simulink model "case5"  (R2024b)
settings: Solver=FixedStepAuto  StartTime=0  StopTime=1  FixedStep=1e-7  RelTol=1e-3
values from neighbouring files (symbols this model uses):
  SG_D_1_D = 0.01056    [IEEE9_case_parameters.m]    (also in case1_parameters.m; case2_parameters.m; case3_parameters.m; case4_parameters.m)
  SG_D_1_EnableSaturation = 0    [IEEE9_case_parameters.m]    (also in case1_parameters.m; case2_parameters.m; case3_parameters.m; case4_parameters.m)
  SG_D_1_f0 = 60    [IEEE9_case_parameters.m]    (also in case1_parameters.m; case2_parameters.m; case3_parameters.m; case4_parameters.m)
  SG_D_1_H = 7.5    [IEEE9_case_parameters.m]    (also in case1_parameters.m; case2_parameters.m; case3_parameters.m; case4_parameters.m)
  SG_D_1_K_A = 20    [IEEE9_case_parameters.m]    (also in case1_parameters.m; case2_parameters.m; case3_parameters.m; case4_parameters.m)
  SG_D_1_K_E = 1.000000e+1    (= 10)    [IEEE9_case_parameters.m]    (also in case1_parameters.m; case2_parameters.m; case3_parameters.m; case4_parameters.m)
  SG_D_1_K_F = 2.363    [IEEE9_case_parameters.m]    (also in case1_parameters.m; case2_parameters.m; case3_parameters.m; case4_parameters.m)
  SG_D_1_K_s = 0.5    [IEEE9_case_parameters.m]    (also in case1_parameters.m = 5; case2_parameters.m = 5; case3_parameters.m = 5; case4_parameters.m = 5)
  SG_D_1_R_a = 0.001088    [IEEE9_case_parameters.m]    (also in case1_parameters.m; case2_parameters.m; case3_parameters.m; case4_parameters.m)
  SG_D_1_S_A = 1    [IEEE9_case_parameters.m]    (also in case1_parameters.m; case2_parameters.m; case3_parameters.m; case4_parameters.m)
  SG_D_1_S_B = 0.103    [IEEE9_case_parameters.m]    (also in case1_parameters.m; case2_parameters.m; case3_parameters.m; case4_parameters.m)
  SG_D_1_S_N = 10.659857    [IEEE9_case_parameters.m]    (also in case1_parameters.m; case2_parameters.m; case3_parameters.m; case4_parameters.m)
  SG_D_1_SpeedPara = 200    [IEEE9_case_parameters.m]    (also in case1_parameters.m; case2_parameters.m; case3_parameters.m; case4_parameters.m)
  SG_D_1_T_0 = 0.720173    [IEEE9_case_parameters.m]    (also in case1_parameters.m = 0.755522; case2_parameters.m = 0.808931; case3_parameters.m = 0.869402; case4_parameters.m = 0.729316)
  SG_D_1_T_1 = 0.3    [IEEE9_case_parameters.m]    (also in case1_parameters.m; case2_parameters.m; case3_parameters.m; case4_parameters.m)
  SG_D_1_T_2 = 0.05    [IEEE9_case_parameters.m]    (also in case1_parameters.m; case2_parameters.m; case3_parameters.m; case4_parameters.m)
  SG_D_1_T_3 = 0.02    [IEEE9_case_parameters.m]    (also in case1_parameters.m; case2_parameters.m; case3_parameters.m; case4_parameters.m)
  SG_D_1_T_4 = 0.005    [IEEE9_case_parameters.m]    (also in case1_parameters.m; case2_parameters.m; case3_parameters.m; case4_parameters.m)
  SG_D_1_T_A = 0.02    [IEEE9_case_parameters.m]    (also in case1_parameters.m; case2_parameters.m; case3_parameters.m; case4_parameters.m)
  SG_D_1_T_dd = 8.000000e+0    (= 8)    [IEEE9_case_parameters.m]    (also in case1_parameters.m; case2_parameters.m; case3_parameters.m; case4_parameters.m)
  SG_D_1_T_ddd = 0.04    [IEEE9_case_parameters.m]    (also in case1_parameters.m; case2_parameters.m; case3_parameters.m; case4_parameters.m)
  SG_D_1_T_E = 0.314    [IEEE9_case_parameters.m]    (also in case1_parameters.m; case2_parameters.m; case3_parameters.m; case4_parameters.m)
  SG_D_1_T_F = 0.35    [IEEE9_case_parameters.m]    (also in case1_parameters.m; case2_parameters.m; case3_parameters.m; case4_parameters.m)
  SG_D_1_T_qd = 0.8    [IEEE9_case_parameters.m]    (also in case1_parameters.m; case2_parameters.m; case3_parameters.m; case4_parameters.m)
  SG_D_1_T_qdd = 0.02    [IEEE9_case_parameters.m]    (also in case1_parameters.m; case2_parameters.m; case3_parameters.m; case4_parameters.m)
  SG_D_1_T_speed = 0.1    [IEEE9_case_parameters.m]    (also in case1_parameters.m = 200; case2_parameters.m = 200; case3_parameters.m = 200; case4_parameters.m = 200)
  SG_D_1_T_w = 0.5    [IEEE9_case_parameters.m]    (also in case1_parameters.m; case2_parameters.m; case3_parameters.m; case4_parameters.m)
  SG_D_1_V_ref = 1.990276    [IEEE9_case_parameters.m]    (also in case1_parameters.m = 2.042296; case2_parameters.m = 2.051388; case3_parameters.m = 2.089584; case4_parameters.m = 2.01845)
  SG_D_1_w_ref = 376.991118    [IEEE9_case_parameters.m]    (also in case1_parameters.m; case2_parameters.m; case3_parameters.m; case4_parameters.m)
  SG_D_1_wb = 6.000000e+1    (= 60)    [IEEE9_case_parameters.m]    (also in case1_parameters.m; case2_parameters.m; case3_parameters.m; case4_parameters.m)
  SG_D_1_x_d = 1.9    [IEEE9_case_parameters.m]    (also in case1_parameters.m; case2_parameters.m; case3_parameters.m; case4_parameters.m)
  SG_D_1_x_dd = 0.302    [IEEE9_case_parameters.m]    (also in case1_parameters.m; case2_parameters.m; case3_parameters.m; case4_parameters.m)
  SG_D_1_x_ddd = 0.204    [IEEE9_case_parameters.m]    (also in case1_parameters.m; case2_parameters.m; case3_parameters.m; case4_parameters.m)
  SG_D_1_x_l = 0.05    [IEEE9_case_parameters.m]    (also in case1_parameters.m; case2_parameters.m; case3_parameters.m; case4_parameters.m)
  SG_D_1_x_q = 1.3    [IEEE9_case_parameters.m]    (also in case1_parameters.m; case2_parameters.m; case3_parameters.m; case4_parameters.m)
  SG_D_1_x_qd = 0.5    [IEEE9_case_parameters.m]    (also in case1_parameters.m; case2_parameters.m; case3_parameters.m; case4_parameters.m)
  SG_D_1_x_qdd = 0.3    [IEEE9_case_parameters.m]    (also in case1_parameters.m; case2_parameters.m; case3_parameters.m; case4_parameters.m)
  SG_D_2_D = 0.02    [IEEE9_case_parameters.m]    (also in case1_parameters.m; case2_parameters.m; case3_parameters.m; case4_parameters.m)
  SG_D_2_EnableSaturation = 0    [IEEE9_case_parameters.m]    (also in case1_parameters.m; case2_parameters.m; case3_parameters.m; case4_parameters.m)
  SG_D_2_f0 = 60    [IEEE9_case_parameters.m]    (also in case1_parameters.m; case2_parameters.m; case3_parameters.m; case4_parameters.m)
  SG_D_2_H = 8.000000e+0    (= 8)    [IEEE9_case_parameters.m]    (also in case1_parameters.m; case2_parameters.m; case3_parameters.m; case4_parameters.m)
  SG_D_2_K_A = 20    [IEEE9_case_parameters.m]    (also in case1_parameters.m; case2_parameters.m; case3_parameters.m; case4_parameters.m)
  SG_D_2_K_E = 1.000000e+1    (= 10)    [IEEE9_case_parameters.m]    (also in case1_parameters.m; case2_parameters.m; case3_parameters.m; case4_parameters.m)
  SG_D_2_K_F = 2.363    [IEEE9_case_parameters.m]    (also in case1_parameters.m; case2_parameters.m; case3_parameters.m; case4_parameters.m)
  SG_D_2_K_s = 0.5    [IEEE9_case_parameters.m]    (also in case1_parameters.m = 4; case2_parameters.m = 4; case3_parameters.m = 4; case4_parameters.m = 4)
  SG_D_2_R_a = 0.001088    [IEEE9_case_parameters.m]    (also in case1_parameters.m; case2_parameters.m; case3_parameters.m; case4_parameters.m)
  SG_D_2_S_A = 1    [IEEE9_case_parameters.m]    (also in case1_parameters.m; case2_parameters.m; case3_parameters.m; case4_parameters.m)
  SG_D_2_S_B = 0.103    [IEEE9_case_parameters.m]    (also in case1_parameters.m; case2_parameters.m; case3_parameters.m; case4_parameters.m)
  SG_D_2_S_N = 10.659857    [IEEE9_case_parameters.m]    (also in case1_parameters.m; case2_parameters.m; case3_parameters.m; case4_parameters.m)
  SG_D_2_SpeedPara = 200    [IEEE9_case_parameters.m]    (also in case1_parameters.m; case2_parameters.m; case3_parameters.m; case4_parameters.m)
  SG_D_2_T_0 = 1.632913    [IEEE9_case_parameters.m]    (also in case1_parameters.m = 1.632925; case2_parameters.m = 1.632915; case3_parameters.m = 1.632914; case4_parameters.m = 1.632927)
  SG_D_2_T_1 = 0.2    [IEEE9_case_parameters.m]    (also in case1_parameters.m; case2_parameters.m; case3_parameters.m; case4_parameters.m)
  SG_D_2_T_2 = 0.05    [IEEE9_case_parameters.m]    (also in case1_parameters.m; case2_parameters.m; case3_parameters.m; case4_parameters.m)
  SG_D_2_T_3 = 0.02    [IEEE9_case_parameters.m]    (also in case1_parameters.m; case2_parameters.m; case3_parameters.m; case4_parameters.m)
  SG_D_2_T_4 = 0.005    [IEEE9_case_parameters.m]    (also in case1_parameters.m; case2_parameters.m; case3_parameters.m; case4_parameters.m)
  SG_D_2_T_A = 0.02    [IEEE9_case_parameters.m]    (also in case1_parameters.m; case2_parameters.m; case3_parameters.m; case4_parameters.m)
  SG_D_2_T_dd = 7.9    [IEEE9_case_parameters.m]    (also in case1_parameters.m; case2_parameters.m; case3_parameters.m; case4_parameters.m)
  SG_D_2_T_ddd = 0.04    [IEEE9_case_parameters.m]    (also in case1_parameters.m; case2_parameters.m; case3_parameters.m; case4_parameters.m)
  SG_D_2_T_E = 0.314    [IEEE9_case_parameters.m]    (also in case1_parameters.m; case2_parameters.m; case3_parameters.m; case4_parameters.m)
  SG_D_2_T_F = 0.35    [IEEE9_case_parameters.m]    (also in case1_parameters.m; case2_parameters.m; case3_parameters.m; case4_parameters.m)
  SG_D_2_T_qd = 0.8    [IEEE9_case_parameters.m]    (also in case1_parameters.m; case2_parameters.m; case3_parameters.m; case4_parameters.m)
  SG_D_2_T_qdd = 0.015    [IEEE9_case_parameters.m]    (also in case1_parameters.m; case2_parameters.m; case3_parameters.m; case4_parameters.m)
  SG_D_2_T_speed = 0.1    [IEEE9_case_parameters.m]    (also in case1_parameters.m = 150; case2_parameters.m = 150; case3_parameters.m = 150; case4_parameters.m = 150)
  SG_D_2_T_w = 0.35    [IEEE9_case_parameters.m]    (also in case1_parameters.m; case2_parameters.m; case3_parameters.m; case4_parameters.m)
  SG_D_2_V_ref = 2.58547    [IEEE9_case_parameters.m]    (also in case1_parameters.m = 2.597896; case2_parameters.m = 2.587136; case3_parameters.m = 2.586042; case4_parameters.m = 2.599679)
  SG_D_2_w_ref = 376.991118    [IEEE9_case_parameters.m]    (also in case1_parameters.m; case2_parameters.m; case3_parameters.m; case4_parameters.m)
  SG_D_2_wb = 6.000000e+1    (= 60)    [IEEE9_case_parameters.m]    (also in case1_parameters.m; case2_parameters.m; case3_parameters.m; case4_parameters.m)
  SG_D_2_x_d = 1.8    [IEEE9_case_parameters.m]    (also in case1_parameters.m; case2_parameters.m; case3_parameters.m; case4_parameters.m)
  SG_D_2_x_dd = 0.302    [IEEE9_case_parameters.m]    (also in case1_parameters.m; case2_parameters.m; case3_parameters.m; case4_parameters.m)
  SG_D_2_x_ddd = 0.204    [IEEE9_case_parameters.m]    (also in case1_parameters.m; case2_parameters.m; case3_parameters.m; case4_parameters.m)
  SG_D_2_x_l = 0.05    [IEEE9_case_parameters.m]    (also in case1_parameters.m; case2_parameters.m; case3_parameters.m; case4_parameters.m)
  SG_D_2_x_q = 1.25    [IEEE9_case_parameters.m]    (also in case1_parameters.m; case2_parameters.m; case3_parameters.m; case4_parameters.m)
  SG_D_2_x_qd = 0.5    [IEEE9_case_parameters.m]    (also in case1_parameters.m; case2_parameters.m; case3_parameters.m; case4_parameters.m)
  SG_D_2_x_qdd = 0.3    [IEEE9_case_parameters.m]    (also in case1_parameters.m; case2_parameters.m; case3_parameters.m; case4_parameters.m)
  SG_D_3_D = 0.02    [IEEE9_case_parameters.m]    (also in case1_parameters.m; case2_parameters.m; case3_parameters.m; case4_parameters.m)
  SG_D_3_EnableSaturation = 0    [IEEE9_case_parameters.m]    (also in case1_parameters.m; case2_parameters.m; case3_parameters.m; case4_parameters.m)
  SG_D_3_f0 = 60    [IEEE9_case_parameters.m]    (also in case1_parameters.m; case2_parameters.m; case3_parameters.m; case4_parameters.m)
  SG_D_3_H = 7.7    [IEEE9_case_parameters.m]    (also in case1_parameters.m; case2_parameters.m; case3_parameters.m; case4_parameters.m)
  SG_D_3_K_A = 20    [IEEE9_case_parameters.m]    (also in case1_parameters.m; case2_parameters.m; case3_parameters.m; case4_parameters.m)
  SG_D_3_K_E = 1.000000e+1    (= 10)    [IEEE9_case_parameters.m]    (also in case1_parameters.m; case2_parameters.m; case3_parameters.m; case4_parameters.m)
  SG_D_3_K_F = 2.363    [IEEE9_case_parameters.m]    (also in case1_parameters.m; case2_parameters.m; case3_parameters.m; case4_parameters.m)
  SG_D_3_K_s = 0.2    [IEEE9_case_parameters.m]    (also in case1_parameters.m = 2; case2_parameters.m = 2; case3_parameters.m = 2; case4_parameters.m = 2)
  SG_D_3_R_a = 0.001088    [IEEE9_case_parameters.m]    (also in case1_parameters.m; case2_parameters.m; case3_parameters.m; case4_parameters.m)
  SG_D_3_S_A = 1    [IEEE9_case_parameters.m]    (also in case1_parameters.m; case2_parameters.m; case3_parameters.m; case4_parameters.m)
  SG_D_3_S_B = 0.103    [IEEE9_case_parameters.m]    (also in case1_parameters.m; case2_parameters.m; case3_parameters.m; case4_parameters.m)
  SG_D_3_S_N = 10.659857    [IEEE9_case_parameters.m]    (also in case1_parameters.m; case2_parameters.m; case3_parameters.m; case4_parameters.m)
  SG_D_3_SpeedPara = 200    [IEEE9_case_parameters.m]    (also in case1_parameters.m; case2_parameters.m; case3_parameters.m; case4_parameters.m)
  SG_D_3_T_0 = 0.850788    [IEEE9_case_parameters.m]    (also in case1_parameters.m = 0.850786; case2_parameters.m = 0.850787; case3_parameters.m; case4_parameters.m = 0.850786)
  SG_D_3_T_1 = 0.2    [IEEE9_case_parameters.m]    (also in case1_parameters.m; case2_parameters.m; case3_parameters.m; case4_parameters.m)
  SG_D_3_T_2 = 0.05    [IEEE9_case_parameters.m]    (also in case1_parameters.m; case2_parameters.m; case3_parameters.m; case4_parameters.m)
  SG_D_3_T_3 = 0.02    [IEEE9_case_parameters.m]    (also in case1_parameters.m; case2_parameters.m; case3_parameters.m; case4_parameters.m)
  SG_D_3_T_4 = 0.005    [IEEE9_case_parameters.m]    (also in case1_parameters.m; case2_parameters.m; case3_parameters.m; case4_parameters.m)
  SG_D_3_T_A = 0.02    [IEEE9_case_parameters.m]    (also in case1_parameters.m; case2_parameters.m; case3_parameters.m; case4_parameters.m)
  SG_D_3_T_dd = 8.1    [IEEE9_case_parameters.m]    (also in case1_parameters.m; case2_parameters.m; case3_parameters.m; case4_parameters.m)
  SG_D_3_T_ddd = 0.04    [IEEE9_case_parameters.m]    (also in case1_parameters.m; case2_parameters.m; case3_parameters.m; case4_parameters.m)
  SG_D_3_T_E = 0.314    [IEEE9_case_parameters.m]    (also in case1_parameters.m; case2_parameters.m; case3_parameters.m; case4_parameters.m)
  SG_D_3_T_F = 0.35    [IEEE9_case_parameters.m]    (also in case1_parameters.m; case2_parameters.m; case3_parameters.m; case4_parameters.m)
  SG_D_3_T_qd = 0.8    [IEEE9_case_parameters.m]    (also in case1_parameters.m; case2_parameters.m; case3_parameters.m; case4_parameters.m)
  SG_D_3_T_qdd = 0.015    [IEEE9_case_parameters.m]    (also in case1_parameters.m; case2_parameters.m; case3_parameters.m; case4_parameters.m)
  SG_D_3_T_speed = 0.1    [IEEE9_case_parameters.m]    (also in case1_parameters.m = 180; case2_parameters.m = 180; case3_parameters.m = 180; case4_parameters.m = 180)
  SG_D_3_T_w = 0.4    [IEEE9_case_parameters.m]    (also in case1_parameters.m; case2_parameters.m; case3_parameters.m; case4_parameters.m)
  SG_D_3_V_ref = 1.892727    [IEEE9_case_parameters.m]    (also in case1_parameters.m = 1.906439; case2_parameters.m = 1.895535; case3_parameters.m = 1.892105; case4_parameters.m = 1.906598)
  SG_D_3_w_ref = 376.991118    [IEEE9_case_parameters.m]    (also in case1_parameters.m; case2_parameters.m; case3_parameters.m; case4_parameters.m)
  SG_D_3_wb = 6.000000e+1    (= 60)    [IEEE9_case_parameters.m]    (also in case1_parameters.m; case2_parameters.m; case3_parameters.m; case4_parameters.m)
  SG_D_3_x_d = 1.85    [IEEE9_case_parameters.m]    (also in case1_parameters.m; case2_parameters.m; case3_parameters.m; case4_parameters.m)
  SG_D_3_x_dd = 0.302    [IEEE9_case_parameters.m]    (also in case1_parameters.m; case2_parameters.m; case3_parameters.m; case4_parameters.m)
  SG_D_3_x_ddd = 0.204    [IEEE9_case_parameters.m]    (also in case1_parameters.m; case2_parameters.m; case3_parameters.m; case4_parameters.m)
  SG_D_3_x_l = 0.05    [IEEE9_case_parameters.m]    (also in case1_parameters.m; case2_parameters.m; case3_parameters.m; case4_parameters.m)
  SG_D_3_x_q = 1.2    [IEEE9_case_parameters.m]    (also in case1_parameters.m; case2_parameters.m; case3_parameters.m; case4_parameters.m)
  SG_D_3_x_qd = 0.5    [IEEE9_case_parameters.m]    (also in case1_parameters.m; case2_parameters.m; case3_parameters.m; case4_parameters.m)
  SG_D_3_x_qdd = 0.3    [IEEE9_case_parameters.m]    (also in case1_parameters.m; case2_parameters.m; case3_parameters.m; case4_parameters.m)
(part 1 of 12)
settings Model: Creator=Greg  LastModifiedBy=Greg

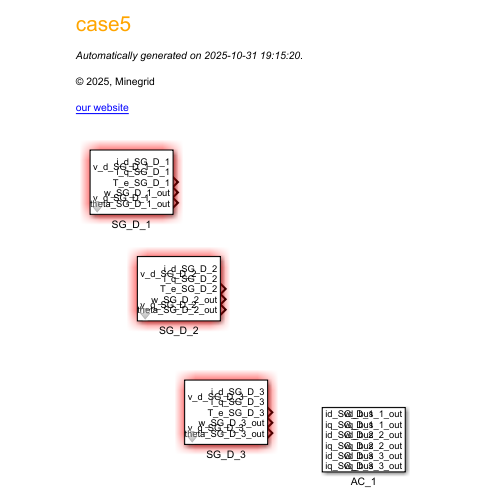
[thumbnail: Simulink's stored preview of the top-level diagram]
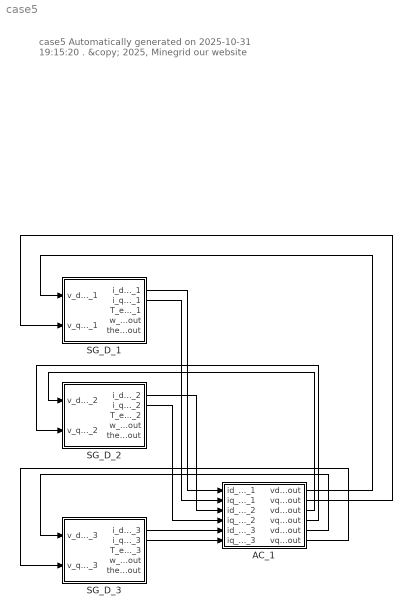
== system case5 ==
  note: case5
      | Automatically generated on 2025-10-31 19:15:20 .
      | &copy; 2025, Minegrid
      | our website
  AC_1 : Subsystem  mask(AC_1){}
      mask help: Parameters Interface of AC_1
  SG_D_1 : Subsystem  mask(SG_D_1){T_0=SG_D_1_T_0, w_ref=SG_D_1_w_ref, V_ref=SG_D_1_V_ref, x_d=SG_D_1_x_d, x_dd=SG_D_1_x_dd, x_ddd=SG_D_1_x_ddd, x_q=SG_D_1_x_q, x_qd=SG_D_1_x_qd, x_qdd=SG_D_1_x_qdd, x_l=SG_D_1_x_l, R_a=SG_D_1_R_a, T_dd=SG_D_1_T_dd, T_ddd=SG_D_1_T_ddd, T_qd=SG_D_1_T_qd, T_qdd=SG_D_1_T_qdd, H=SG_D_1_H, D=SG_D_1_D, SpeedPara=SG_D_1_SpeedPara, K_A=SG_D_1_K_A, EnableSaturation=SG_D_1_EnableSaturation, f0=SG_D_1_f0, T_speed=SG_D_1_T_speed, T_E=SG_D_1_T_E, T_A=SG_D_1_T_A, T_F=SG_D_1_T_F, K_E=SG_D_1_K_E, K_F=SG_D_1_K_F, K_s=SG_D_1_K_s, T_1=SG_D_1_T_1, T_2=SG_D_1_T_2, T_3=SG_D_1_T_3, T_4=SG_D_1_T_4, T_w=SG_D_1_T_w, wb=SG_D_1_wb, S_A=SG_D_1_S_A, S_B=SG_D_1_S_B, S_N=SG_D_1_S_N}
      mask help: Parameters Interface of SG_D_1
  SG_D_2 : Subsystem  mask(SG_D_2){T_0=SG_D_2_T_0, w_ref=SG_D_2_w_ref, V_ref=SG_D_2_V_ref, x_d=SG_D_2_x_d, x_dd=SG_D_2_x_dd, x_ddd=SG_D_2_x_ddd, x_q=SG_D_2_x_q, x_qd=SG_D_2_x_qd, x_qdd=SG_D_2_x_qdd, x_l=SG_D_2_x_l, R_a=SG_D_2_R_a, T_dd=SG_D_2_T_dd, T_ddd=SG_D_2_T_ddd, T_qd=SG_D_2_T_qd, T_qdd=SG_D_2_T_qdd, H=SG_D_2_H, D=SG_D_2_D, SpeedPara=SG_D_2_SpeedPara, K_A=SG_D_2_K_A, EnableSaturation=SG_D_2_EnableSaturation, f0=SG_D_2_f0, T_speed=SG_D_2_T_speed, T_E=SG_D_2_T_E, T_A=SG_D_2_T_A, T_F=SG_D_2_T_F, K_E=SG_D_2_K_E, K_F=SG_D_2_K_F, K_s=SG_D_2_K_s, T_1=SG_D_2_T_1, T_2=SG_D_2_T_2, T_3=SG_D_2_T_3, T_4=SG_D_2_T_4, T_w=SG_D_2_T_w, wb=SG_D_2_wb, S_A=SG_D_2_S_A, S_B=SG_D_2_S_B, S_N=SG_D_2_S_N}
      mask help: Parameters Interface of SG_D_2
  SG_D_3 : Subsystem  mask(SG_D_3){T_0=SG_D_3_T_0, w_ref=SG_D_3_w_ref, V_ref=SG_D_3_V_ref, x_d=SG_D_3_x_d, x_dd=SG_D_3_x_dd, x_ddd=SG_D_3_x_ddd, x_q=SG_D_3_x_q, x_qd=SG_D_3_x_qd, x_qdd=SG_D_3_x_qdd, x_l=SG_D_3_x_l, R_a=SG_D_3_R_a, T_dd=SG_D_3_T_dd, T_ddd=SG_D_3_T_ddd, T_qd=SG_D_3_T_qd, T_qdd=SG_D_3_T_qdd, H=SG_D_3_H, D=SG_D_3_D, SpeedPara=SG_D_3_SpeedPara, K_A=SG_D_3_K_A, EnableSaturation=SG_D_3_EnableSaturation, f0=SG_D_3_f0, T_speed=SG_D_3_T_speed, T_E=SG_D_3_T_E, T_A=SG_D_3_T_A, T_F=SG_D_3_T_F, K_E=SG_D_3_K_E, K_F=SG_D_3_K_F, K_s=SG_D_3_K_s, T_1=SG_D_3_T_1, T_2=SG_D_3_T_2, T_3=SG_D_3_T_3, T_4=SG_D_3_T_4, T_w=SG_D_3_T_w, wb=SG_D_3_wb, S_A=SG_D_3_S_A, S_B=SG_D_3_S_B, S_N=SG_D_3_S_N}
      mask help: Parameters Interface of SG_D_3
  wires:
  SG_D_2/2(i_q_SG_D_2) -> AC_1/4(iq_SG_D_2)
  SG_D_1/2(i_q_SG_D_1) -> AC_1/2(iq_SG_D_1)
  SG_D_1/1(i_d_SG_D_1) -> AC_1/1(id_SG_D_1)
  SG_D_2/1(i_d_SG_D_2) -> AC_1/3(id_SG_D_2)
  AC_1/1(vd_bus_1_out) -> SG_D_1/1(v_d_SG_D_1)
  SG_D_3/1(i_d_SG_D_3) -> AC_1/5(id_SG_D_3)
  AC_1/2(vq_bus_1_out) -> SG_D_1/2(v_q_SG_D_1)
  SG_D_3/2(i_q_SG_D_3) -> AC_1/6(iq_SG_D_3)
  AC_1/3(vd_bus_2_out) -> SG_D_2/1(v_d_SG_D_2)
  AC_1/4(vq_bus_2_out) -> SG_D_2/2(v_q_SG_D_2)
  AC_1/5(vd_bus_3_out) -> SG_D_3/1(v_d_SG_D_3)
  AC_1/6(vq_bus_3_out) -> SG_D_3/2(v_q_SG_D_3)

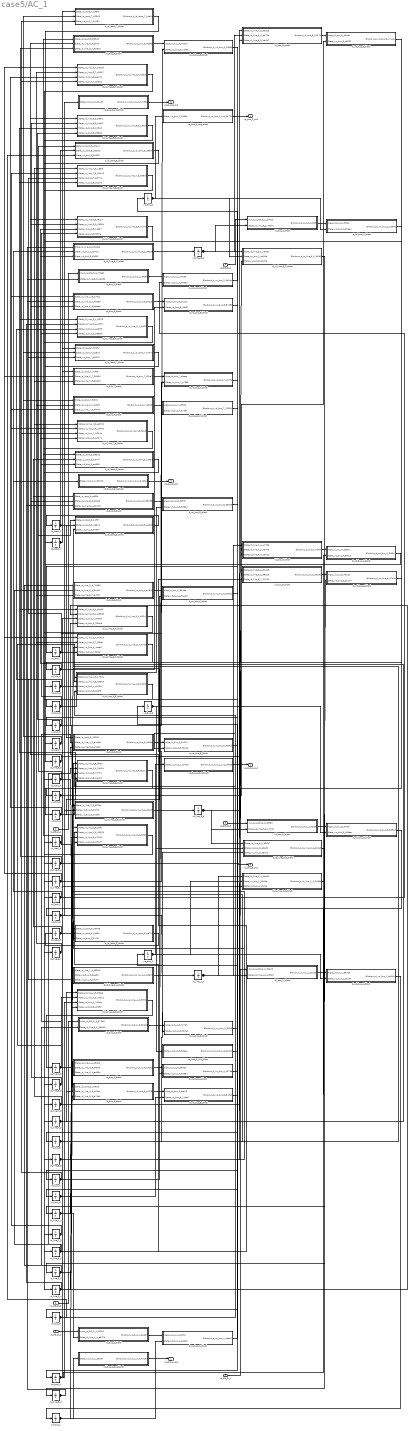
== system case5/AC_1 ==
  id_SG_D_1 : Inport
  iq_SG_D_1 : Inport  Port=2
  id_SG_D_2 : Inport  Port=3
  iq_SG_D_2 : Inport  Port=4
  id_SG_D_3 : Inport  Port=5
  iq_SG_D_3 : Inport  Port=6
  d_id_line_1_4_block : Subsystem
  d_id_line_3_6_block : Subsystem
  d_id_line_4_5_block : Subsystem
  d_id_line_5_6_block : Subsystem
  d_id_line_6_7_block : Subsystem
  d_id_line_7_8_block : Subsystem
  d_id_line_8_2_block : Subsystem
  d_id_line_8_9_block : Subsystem
  d_id_line_9_4_block : Subsystem
  d_id_load_5_block : Subsystem
  d_id_load_7_block : Subsystem
  d_id_load_9_block : Subsystem
  d_iq_line_1_4_block : Subsystem
  d_iq_line_3_6_block : Subsystem
  d_iq_line_4_5_block : Subsystem
  d_iq_line_5_6_block : Subsystem
  d_iq_line_6_7_block : Subsystem
  d_iq_line_7_8_block : Subsystem
  d_iq_line_8_2_block : Subsystem
  d_iq_line_8_9_block : Subsystem
  d_iq_line_9_4_block : Subsystem
  d_iq_load_5_block : Subsystem
  d_iq_load_7_block : Subsystem
  d_iq_load_9_block : Subsystem
  d_vd_bus_1_block : Subsystem
  d_vd_bus_2_block : Subsystem
  d_vd_bus_3_block : Subsystem
  d_vd_bus_4_block : Subsystem
  d_vd_bus_5_block : Subsystem
  d_vd_bus_6_block : Subsystem
  d_vd_bus_7_block : Subsystem
  d_vd_bus_8_block : Subsystem
  d_vd_bus_9_block : Subsystem
  d_vq_bus_1_block : Subsystem
  d_vq_bus_2_block : Subsystem
  d_vq_bus_3_block : Subsystem
  d_vq_bus_4_block : Subsystem
  d_vq_bus_5_block : Subsystem
  d_vq_bus_6_block : Subsystem
  d_vq_bus_7_block : Subsystem
  d_vq_bus_8_block : Subsystem
  d_vq_bus_9_block : Subsystem
  id_bus_1_block : Subsystem
  id_bus_2_block : Subsystem
  id_bus_3_block : Subsystem
  id_bus_4_block : Subsystem
  id_bus_5_block : Subsystem
  id_bus_6_block : Subsystem
  id_bus_7_block : Subsystem
  id_bus_8_block : Subsystem
  id_bus_9_block : Subsystem
  id_line_1_4 : Integrator  InitialCondition=0.6535
  id_line_3_6 : Integrator  InitialCondition=0.8439
  id_line_4_5 : Integrator  InitialCondition=0.2782
  id_line_5_6 : Integrator  InitialCondition=-0.6203
  id_line_6_7 : Integrator  InitialCondition=0.236
  id_line_7_8 : Integrator  InitialCondition=-0.7627
  id_line_8_2 : Integrator  InitialCondition=-1.6328
  id_line_8_9 : Integrator  InitialCondition=0.8876
  id_line_9_4 : Integrator  InitialCondition=-0.3688
  id_load_5 : Integrator  InitialCondition=0.8820374198700516
  id_load_7 : Integrator  InitialCondition=1.0024523883976943
  id_load_9 : Integrator  InitialCondition=1.240018118653886
  iq_bus_1_block : Subsystem
  iq_bus_2_block : Subsystem
  iq_bus_3_block : Subsystem
  iq_bus_4_block : Subsystem
  iq_bus_5_block : Subsystem
  iq_bus_6_block : Subsystem
  iq_bus_7_block : Subsystem
  iq_bus_8_block : Subsystem
  iq_bus_9_block : Subsystem
  iq_line_1_4 : Integrator  InitialCondition=-0.2504
  iq_line_3_6 : Integrator  InitialCondition=0.1043
  iq_line_4_5 : Integrator  InitialCondition=-0.0879
  iq_line_5_6 : Integrator  InitialCondition=0.0348
  iq_line_6_7 : Integrator  InitialCondition=-0.1449
  iq_line_7_8 : Integrator  InitialCondition=0.0214
  iq_line_8_2 : Integrator  InitialCondition=-0.1355
  iq_line_8_9 : Integrator  InitialCondition=-0.0687
  iq_line_9_4 : Integrator  InitialCondition=0.327
  iq_load_5 : Integrator  InitialCondition=-0.3735355762849134
  iq_load_7 : Integrator  InitialCondition=-0.3424626103057441
  iq_load_9 : Integrator  InitialCondition=-0.6252597675885702
  vd_bus_1 : Integrator  InitialCondition=1.0
  vd_bus_1_out_block : Subsystem
  vd_bus_2 : Integrator  InitialCondition=0.9831295998982378
  vd_bus_2_out_block : Subsystem
  vd_bus_3 : Integrator  InitialCondition=0.9954886816761164
  vd_bus_3_out_block : Subsystem
  vd_bus_4 : Integrator  InitialCondition=0.9850944132545842
  vd_bus_5 : Integrator  InitialCondition=0.9721239885442489
  vd_bus_6 : Integrator  InitialCondition=1.0018067875887238
  vd_bus_7 : Integrator  InitialCondition=0.9839740918091784
  vd_bus_8 : Integrator  InitialCondition=0.9918849362505074
  vd_bus_9 : Integrator  InitialCondition=0.9527792114130469
  vq_bus_1 : Integrator  InitialCondition=0.0
  vq_bus_1_out_block : Subsystem
  vq_bus_2 : Integrator  InitialCondition=0.18291033268771614
  vq_bus_2_out_block : Subsystem
  vq_bus_3 : Integrator  InitialCondition=0.09488037022876668
  vq_bus_3_out_block : Subsystem
  vq_bus_4 : Integrator  InitialCondition=-0.03890158756630978
  vq_bus_5 : Integrator  InitialCondition=-0.06389643762457121
  vq_bus_6 : Integrator  InitialCondition=0.043770445658715566
  vq_bus_7 : Integrator  InitialCondition=0.020865646177209426
  vq_bus_8 : Integrator  InitialCondition=0.07744433881790898
  vq_bus_9 : Integrator  InitialCondition=-0.06811306352767708
  vd_bus_1_out : Outport
  vq_bus_1_out : Outport  Port=2
  vd_bus_2_out : Outport  Port=3
  vq_bus_2_out : Outport  Port=4
  vd_bus_3_out : Outport  Port=5
  vq_bus_3_out : Outport  Port=6
  wires:
  id_line_4_5/1 -> d_id_line_4_5_block/1(State_id_line_4_5_17bd4), d_iq_line_4_5_block/1(State_id_line_4_5_5fe62), id_bus_4_block/2(State_id_line_4_5_4344a), id_bus_5_block/2(State_id_line_4_5_425cc)
  id_bus_6_block/1(Blockout_id_bus_6_b6b8c) -> d_vd_bus_6_block/1(Alge_id_bus_6_4022d)
  d_iq_line_1_4_block/1(Blockout_d_iq_line_1_4_2dd06) -> iq_line_1_4/1
  id_line_6_7/1 -> id_bus_6_block/3(State_id_line_6_7_21130), d_id_line_6_7_block/1(State_id_line_6_7_b019b), id_bus_7_block/2(State_id_line_6_7_06d30), d_iq_line_6_7_block/1(State_id_line_6_7_0d433)
  id_bus_2_block/1(Blockout_id_bus_2_c40f0) -> d_vd_bus_2_block/1(Alge_id_bus_2_9f42b)
  iq_bus_4_block/1(Blockout_iq_bus_4_10eb1) -> d_vq_bus_4_block/1(Alge_iq_bus_4_d306c)
  iq_SG_D_2/1 -> iq_bus_2_block/1(Input_iq_SG_D_2_79eaf)
  vq_bus_2_out_block/1(Blockout_vq_bus_2_out_5d720) -> vq_bus_2_out/1
  d_id_line_1_4_block/1(Blockout_d_id_line_1_4_69e37) -> id_line_1_4/1
  iq_SG_D_3/1 -> iq_bus_3_block/1(Input_iq_SG_D_3_679b5)
  iq_bus_5_block/1(Blockout_iq_bus_5_0fe3b) -> d_vq_bus_5_block/1(Alge_iq_bus_5_3167d)
  d_iq_line_8_2_block/1(Blockout_d_iq_line_8_2_50cf1) -> iq_line_8_2/1
  id_SG_D_3/1 -> id_bus_3_block/1(Input_id_SG_D_3_99f83)
  d_vd_bus_4_block/1(Blockout_d_vd_bus_4_f5d06) -> vd_bus_4/1
  vd_bus_3_out_block/1(Blockout_vd_bus_3_out_7cfd2) -> vd_bus_3_out/1
  d_iq_line_4_5_block/1(Blockout_d_iq_line_4_5_957bf) -> iq_line_4_5/1
  id_bus_4_block/1(Blockout_id_bus_4_70fca) -> d_vd_bus_4_block/1(Alge_id_bus_4_3c99c)
  vd_bus_1_out_block/1(Blockout_vd_bus_1_out_40167) -> vd_bus_1_out/1
  vq_bus_1_out_block/1(Blockout_vq_bus_1_out_208d9) -> vq_bus_1_out/1
  iq_SG_D_1/1 -> iq_bus_1_block/1(Input_iq_SG_D_1_08f14)
  id_bus_9_block/1(Blockout_id_bus_9_60bfe) -> d_vd_bus_9_block/1(Alge_id_bus_9_7e67e)
  iq_load_5/1 -> iq_bus_5_block/1(State_iq_load_5_13280), d_id_load_5_block/2(State_iq_load_5_a5206), d_iq_load_5_block/2(State_iq_load_5_4667a)
  iq_line_7_8/1 -> d_iq_line_7_8_block/2(State_iq_line_7_8_38443), iq_bus_7_block/3(State_iq_line_7_8_6f400), d_id_line_7_8_block/2(State_iq_line_7_8_154d0), iq_bus_8_block/1(State_iq_line_7_8_27acc)
  id_SG_D_2/1 -> id_bus_2_block/1(Input_id_SG_D_2_cb453)
  id_SG_D_1/1 -> id_bus_1_block/1(Input_id_SG_D_1_9c228)
  iq_bus_9_block/1(Blockout_iq_bus_9_35095) -> d_vq_bus_9_block/1(Alge_iq_bus_9_3d507)
  vq_bus_3_out_block/1(Blockout_vq_bus_3_out_e2cb2) -> vq_bus_3_out/1
  iq_bus_8_block/1(Blockout_iq_bus_8_30cc3) -> d_vq_bus_8_block/1(Alge_iq_bus_8_1b1c2)
  iq_line_5_6/1 -> d_id_line_5_6_block/2(State_iq_line_5_6_2c004), d_iq_line_5_6_block/2(State_iq_line_5_6_03329), iq_bus_5_block/3(State_iq_line_5_6_a1b62), iq_bus_6_block/2(State_iq_line_5_6_5b4f1)
  id_bus_3_block/1(Blockout_id_bus_3_bec8f) -> d_vd_bus_3_block/1(Alge_id_bus_3_04cef)
  id_bus_8_block/1(Blockout_id_bus_8_10175) -> d_vd_bus_8_block/1(Alge_id_bus_8_d2bcb)
  iq_bus_7_block/1(Blockout_iq_bus_7_c0ccf) -> d_vq_bus_7_block/1(Alge_iq_bus_7_45bb2)
  d_vd_bus_1_block/1(Blockout_d_vd_bus_1_cb049) -> vd_bus_1/1
  vd_bus_2/1 -> d_vq_bus_2_block/2(State_vd_bus_2_003ed), vd_bus_2_out_block/1(State_vd_bus_2_9b70b), d_id_line_8_2_block/2(State_vd_bus_2_be716)
  vd_bus_6/1 -> d_vq_bus_6_block/2(State_vd_bus_6_96a25), d_id_line_3_6_block/3(State_vd_bus_6_aaa66), d_id_line_5_6_block/4(State_vd_bus_6_16423), d_id_line_6_7_block/3(State_vd_bus_6_ae47b)
  iq_bus_2_block/1(Blockout_iq_bus_2_efb5b) -> d_vq_bus_2_block/1(Alge_iq_bus_2_b4b58)
  d_vq_bus_8_block/1(Blockout_d_vq_bus_8_57dfd) -> vq_bus_8/1
  iq_line_4_5/1 -> d_iq_line_4_5_block/2(State_iq_line_4_5_78122), iq_bus_4_block/2(State_iq_line_4_5_0f8d8), iq_bus_5_block/2(State_iq_line_4_5_a44be), d_id_line_4_5_block/2(State_iq_line_4_5_655b9)
  d_iq_line_8_9_block/1(Blockout_d_iq_line_8_9_1ed33) -> iq_line_8_9/1
  id_line_9_4/1 -> id_bus_4_block/3(State_id_line_9_4_2502b), d_id_line_9_4_block/1(State_id_line_9_4_837f3), id_bus_9_block/3(State_id_line_9_4_83515), d_iq_line_9_4_block/1(State_id_line_9_4_c3c0d)
  vq_bus_8/1 -> d_iq_line_8_2_block/3(State_vq_bus_8_a1826), d_iq_line_7_8_block/4(State_vq_bus_8_202ba), d_iq_line_8_9_block/3(State_vq_bus_8_b13ad), d_vd_bus_8_block/2(State_vq_bus_8_c6552)
  vd_bus_4/1 -> d_id_line_1_4_block/3(State_vd_bus_4_1db4d), d_id_line_9_4_block/3(State_vd_bus_4_e4399), d_id_line_4_5_block/3(State_vd_bus_4_6c299), d_vq_bus_4_block/2(State_vd_bus_4_b3884)
  iq_load_7/1 -> d_id_load_7_block/2(State_iq_load_7_60963), d_iq_load_7_block/2(State_iq_load_7_a25bd), iq_bus_7_block/1(State_iq_load_7_fc531)
  id_bus_7_block/1(Blockout_id_bus_7_23be7) -> d_vd_bus_7_block/1(Alge_id_bus_7_c0ece)
  iq_line_9_4/1 -> d_id_line_9_4_block/2(State_iq_line_9_4_dc97c), iq_bus_4_block/3(State_iq_line_9_4_ed85c), iq_bus_9_block/3(State_iq_line_9_4_06703), d_iq_line_9_4_block/2(State_iq_line_9_4_03835)
  vq_bus_6/1 -> d_vd_bus_6_block/2(State_vq_bus_6_3b173), d_iq_line_3_6_block/3(State_vq_bus_6_39c16), d_iq_line_6_7_block/3(State_vq_bus_6_4ace9), d_iq_line_5_6_block/4(State_vq_bus_6_551df)
  d_id_load_7_block/1(Blockout_d_id_load_7_04e2e) -> id_load_7/1
  iq_bus_6_block/1(Blockout_iq_bus_6_a4840) -> d_vq_bus_6_block/1(Alge_iq_bus_6_9948a)
  d_vd_bus_7_block/1(Blockout_d_vd_bus_7_c07fa) -> vd_bus_7/1
  d_vq_bus_7_block/1(Blockout_d_vq_bus_7_12864) -> vq_bus_7/1
  id_line_5_6/1 -> d_id_line_5_6_block/1(State_id_line_5_6_f0fe5), d_iq_line_5_6_block/1(State_id_line_5_6_8cff1), id_bus_5_block/3(State_id_line_5_6_e79c9), id_bus_6_block/2(State_id_line_5_6_98abd)
  id_bus_5_block/1(Blockout_id_bus_5_e7f75) -> d_vd_bus_5_block/1(Alge_id_bus_5_8ca73)
  iq_bus_3_block/1(Blockout_iq_bus_3_3b6b3) -> d_vq_bus_3_block/1(Alge_iq_bus_3_7b7af)
  id_bus_1_block/1(Blockout_id_bus_1_91a25) -> d_vd_bus_1_block/1(Alge_id_bus_1_8840e)
  iq_bus_1_block/1(Blockout_iq_bus_1_da657) -> d_vq_bus_1_block/1(Alge_iq_bus_1_bc35c)
  vd_bus_2_out_block/1(Blockout_vd_bus_2_out_4bf4d) -> vd_bus_2_out/1
  iq_line_3_6/1 -> d_id_line_3_6_block/1(State_iq_line_3_6_0028c), iq_bus_6_block/1(State_iq_line_3_6_7b556), iq_bus_3_block/2(State_iq_line_3_6_d3a99)
  d_id_line_6_7_block/1(Blockout_d_id_line_6_7_ed3ed) -> id_line_6_7/1
  d_iq_line_9_4_block/1(Blockout_d_iq_line_9_4_b0247) -> iq_line_9_4/1
  d_iq_load_5_block/1(Blockout_d_iq_load_5_ea36b) -> iq_load_5/1
  d_id_line_5_6_block/1(Blockout_d_id_line_5_6_90114) -> id_line_5_6/1
  vd_bus_7/1 -> d_id_load_7_block/3(State_vd_bus_7_34461), d_id_line_6_7_block/4(State_vd_bus_7_eaeb2), d_vq_bus_7_block/2(State_vd_bus_7_3739f), d_id_line_7_8_block/3(State_vd_bus_7_5624b)
  d_id_line_8_2_block/1(Blockout_d_id_line_8_2_55ace) -> id_line_8_2/1
  id_line_3_6/1 -> d_iq_line_3_6_block/1(State_id_line_3_6_990b7), id_bus_6_block/1(State_id_line_3_6_811b8), id_bus_3_block/2(State_id_line_3_6_1713b)
  d_id_line_3_6_block/1(Blockout_d_id_line_3_6_09483) -> id_line_3_6/1
  vq_bus_7/1 -> d_vd_bus_7_block/2(State_vq_bus_7_b7f85), d_iq_line_7_8_block/3(State_vq_bus_7_6977a), d_iq_load_7_block/3(State_vq_bus_7_b5d78), d_iq_line_6_7_block/4(State_vq_bus_7_fbcef)
  iq_line_8_9/1 -> d_id_line_8_9_block/2(State_iq_line_8_9_03554), d_iq_line_8_9_block/2(State_iq_line_8_9_bc607), iq_bus_8_block/3(State_iq_line_8_9_6eee5), iq_bus_9_block/2(State_iq_line_8_9_086c3)
  id_line_8_9/1 -> id_bus_8_block/3(State_id_line_8_9_be4b7), d_id_line_8_9_block/1(State_id_line_8_9_f8c14), d_iq_line_8_9_block/1(State_id_line_8_9_666cc), id_bus_9_block/2(State_id_line_8_9_6f7fd)
  id_line_8_2/1 -> d_iq_line_8_2_block/1(State_id_line_8_2_763ed), id_bus_2_block/2(State_id_line_8_2_49dbc), id_bus_8_block/2(State_id_line_8_2_6b72a)
  iq_line_8_2/1 -> d_id_line_8_2_block/1(State_iq_line_8_2_968c6), iq_bus_2_block/2(State_iq_line_8_2_2ed82), iq_bus_8_block/2(State_iq_line_8_2_45289)
  id_line_7_8/1 -> d_id_line_7_8_block/1(State_id_line_7_8_e67d2), d_iq_line_7_8_block/1(State_id_line_7_8_196fb), id_bus_7_block/3(State_id_line_7_8_80602), id_bus_8_block/1(State_id_line_7_8_30e25)
  vq_bus_9/1 -> d_vd_bus_9_block/2(State_vq_bus_9_1df90), d_iq_load_9_block/3(State_vq_bus_9_617f4), d_iq_line_8_9_block/4(State_vq_bus_9_0596d), d_iq_line_9_4_block/4(State_vq_bus_9_291a8)
  iq_line_6_7/1 -> d_id_line_6_7_block/2(State_iq_line_6_7_c30b7), d_iq_line_6_7_block/2(State_iq_line_6_7_8faef), iq_bus_6_block/3(State_iq_line_6_7_a49c1), iq_bus_7_block/2(State_iq_line_6_7_dc5b1)
  vd_bus_1/1 -> d_vq_bus_1_block/2(State_vd_bus_1_e6515), d_id_line_1_4_block/2(State_vd_bus_1_aee9d), vd_bus_1_out_block/1(State_vd_bus_1_d8d67)
  id_line_1_4/1 -> d_iq_line_1_4_block/1(State_id_line_1_4_b0e34), id_bus_1_block/2(State_id_line_1_4_23de7), id_bus_4_block/1(State_id_line_1_4_47296)
  iq_line_1_4/1 -> d_id_line_1_4_block/1(State_iq_line_1_4_f9009), iq_bus_1_block/2(State_iq_line_1_4_e657d), iq_bus_4_block/1(State_iq_line_1_4_c5db2)
  iq_load_9/1 -> d_id_load_9_block/2(State_iq_load_9_0074f), d_iq_load_9_block/2(State_iq_load_9_0cd3a), iq_bus_9_block/1(State_iq_load_9_e5f0b)
  vd_bus_8/1 -> d_id_line_7_8_block/4(State_vd_bus_8_a9172), d_id_line_8_2_block/3(State_vd_bus_8_d36f6), d_id_line_8_9_block/3(State_vd_bus_8_1c687), d_vq_bus_8_block/2(State_vd_bus_8_d6cf7)
  id_load_9/1 -> d_id_load_9_block/1(State_id_load_9_852e2), d_iq_load_9_block/1(State_id_load_9_b9788), id_bus_9_block/1(State_id_load_9_599d3)
  vd_bus_9/1 -> d_vq_bus_9_block/2(State_vd_bus_9_5d984), d_id_line_8_9_block/4(State_vd_bus_9_9fd7e), d_id_line_9_4_block/4(State_vd_bus_9_b8585), d_id_load_9_block/3(State_vd_bus_9_ae388)
  id_load_7/1 -> d_id_load_7_block/1(State_id_load_7_b98f0), d_iq_load_7_block/1(State_id_load_7_92af4), id_bus_7_block/1(State_id_load_7_7bf08)
  id_load_5/1 -> d_id_load_5_block/1(State_id_load_5_4be11), d_iq_load_5_block/1(State_id_load_5_12f97), id_bus_5_block/1(State_id_load_5_d4ed3)
  vq_bus_2/1 -> d_vd_bus_2_block/2(State_vq_bus_2_626a1), d_iq_line_8_2_block/2(State_vq_bus_2_a450a), vq_bus_2_out_block/1(State_vq_bus_2_2533a)
  vd_bus_5/1 -> d_vq_bus_5_block/2(State_vd_bus_5_f0a26), d_id_load_5_block/3(State_vd_bus_5_53255), d_id_line_4_5_block/4(State_vd_bus_5_8ddf9), d_id_line_5_6_block/3(State_vd_bus_5_7c77b)
  d_id_line_9_4_block/1(Blockout_d_id_line_9_4_0af09) -> id_line_9_4/1
  vq_bus_5/1 -> d_vd_bus_5_block/2(State_vq_bus_5_14cdd), d_iq_load_5_block/3(State_vq_bus_5_ae904), d_iq_line_4_5_block/4(State_vq_bus_5_c2555), d_iq_line_5_6_block/3(State_vq_bus_5_a71a3)
  vq_bus_4/1 -> d_iq_line_1_4_block/3(State_vq_bus_4_12e2c), d_vd_bus_4_block/2(State_vq_bus_4_56f16), d_iq_line_4_5_block/3(State_vq_bus_4_7d2aa), d_iq_line_9_4_block/3(State_vq_bus_4_0a95d)
  vd_bus_3/1 -> d_vq_bus_3_block/2(State_vd_bus_3_f2360), d_id_line_3_6_block/2(State_vd_bus_3_b4f76), vd_bus_3_out_block/1(State_vd_bus_3_3d199)
  vq_bus_3/1 -> d_iq_line_3_6_block/2(State_vq_bus_3_aba8c), d_vd_bus_3_block/2(State_vq_bus_3_406ee), vq_bus_3_out_block/1(State_vq_bus_3_9de4a)
  vq_bus_1/1 -> d_iq_line_1_4_block/2(State_vq_bus_1_10e2e), d_vd_bus_1_block/2(State_vq_bus_1_c0d62), vq_bus_1_out_block/1(State_vq_bus_1_cd4b3)
  d_id_line_4_5_block/1(Blockout_d_id_line_4_5_8120d) -> id_line_4_5/1
  d_id_load_9_block/1(Blockout_d_id_load_9_1c904) -> id_load_9/1
  d_vq_bus_4_block/1(Blockout_d_vq_bus_4_4979a) -> vq_bus_4/1
  d_vq_bus_1_block/1(Blockout_d_vq_bus_1_c9ee7) -> vq_bus_1/1
  d_id_load_5_block/1(Blockout_d_id_load_5_989b8) -> id_load_5/1
  d_iq_line_5_6_block/1(Blockout_d_iq_line_5_6_5852f) -> iq_line_5_6/1
  d_id_line_7_8_block/1(Blockout_d_id_line_7_8_f2a9f) -> id_line_7_8/1
  d_id_line_8_9_block/1(Blockout_d_id_line_8_9_41799) -> id_line_8_9/1
  d_iq_load_9_block/1(Blockout_d_iq_load_9_aa725) -> iq_load_9/1
  d_iq_line_3_6_block/1(Blockout_d_iq_line_3_6_60ca3) -> iq_line_3_6/1
  d_vd_bus_8_block/1(Blockout_d_vd_bus_8_47c26) -> vd_bus_8/1
  d_iq_line_6_7_block/1(Blockout_d_iq_line_6_7_67cbf) -> iq_line_6_7/1
  d_iq_line_7_8_block/1(Blockout_d_iq_line_7_8_896d8) -> iq_line_7_8/1
  d_vq_bus_9_block/1(Blockout_d_vq_bus_9_906de) -> vq_bus_9/1
  d_iq_load_7_block/1(Blockout_d_iq_load_7_b7b7d) -> iq_load_7/1
  d_vq_bus_5_block/1(Blockout_d_vq_bus_5_9d8bd) -> vq_bus_5/1
  d_vd_bus_2_block/1(Blockout_d_vd_bus_2_1e6bd) -> vd_bus_2/1
  d_vd_bus_3_block/1(Blockout_d_vd_bus_3_3d9b3) -> vd_bus_3/1
  d_vq_bus_3_block/1(Blockout_d_vq_bus_3_ffd35) -> vq_bus_3/1
  d_vq_bus_2_block/1(Blockout_d_vq_bus_2_8d2c4) -> vq_bus_2/1
  d_vd_bus_5_block/1(Blockout_d_vd_bus_5_8454f) -> vd_bus_5/1
  d_vd_bus_6_block/1(Blockout_d_vd_bus_6_37b4b) -> vd_bus_6/1
  d_vd_bus_9_block/1(Blockout_d_vd_bus_9_48b9f) -> vd_bus_9/1
  d_vq_bus_6_block/1(Blockout_d_vq_bus_6_aa0b1) -> vq_bus_6/1

== system case5/SG_D_1 ==
  v_d_SG_D_1 : Inport
  v_q_SG_D_1 : Inport  Port=2
  E_fd_SG_D_1 : Integrator  InitialCondition=1.912783795778084
  Px_1_SG_D_1 : Integrator  InitialCondition=0.0
  Px_2_SG_D_1 : Integrator  InitialCondition=0.0
  Px_3_SG_D_1 : Integrator  InitialCondition=1.1814255994905352e-24
  R_f_SG_D_1 : Integrator  InitialCondition=12.91402316978175
  T_e_SG_D_1_block : Subsystem
  T_m_SG_D_1 : Integrator  InitialCondition=0.6540136334844647
  V_f_SG_D_1 : Integrator  InitialCondition=19.127837957780837
  d_E_fd_SG_D_1_block : Subsystem
  d_Px_1_SG_D_1_block : Subsystem
  d_Px_2_SG_D_1_block : Subsystem
  d_Px_3_SG_D_1_block : Subsystem
  d_R_f_SG_D_1_block : Subsystem
  d_T_m_SG_D_1_block : Subsystem
  d_V_f_SG_D_1_block : Subsystem
  d_psi_1d_SG_D_1_block : Subsystem
  d_psi_d_SG_D_1_block : Subsystem
  d_psi_fd_SG_D_1_block : Subsystem
  d_psi_gq_SG_D_1_block : Subsystem
  d_psi_kq_SG_D_1_block : Subsystem
  d_psi_q_SG_D_1_block : Subsystem
  d_theta_SG_D_1_block : Subsystem
  d_w_SG_D_1_block : Subsystem
  i_d_SG_D_1_block : Subsystem
  i_q_SG_D_1_block : Subsystem
  psi_1d_SG_D_1 : Integrator  InitialCondition=0.8707495592836506
  psi_d_SG_D_1 : Integrator  InitialCondition=0.8425864718108279
  psi_fd_SG_D_1 : Integrator  InitialCondition=1.0126915201466762
  psi_gq_SG_D_1 : Integrator  InitialCondition=0.33223394778626014
  psi_kq_SG_D_1 : Integrator  InitialCondition=-0.5191155434160314
  psi_q_SG_D_1 : Integrator  InitialCondition=-0.5398801651526727
  theta_SG_D_1 : Integrator  InitialCondition=0.5695668584576191
  theta_SG_D_1_out_block : Subsystem
  w_SG_D_1 : Integrator  InitialCondition=376.99111843077515
  w_SG_D_1_out_block : Subsystem
  i_d_SG_D_1 : Outport
  i_q_SG_D_1 : Outport  Port=2
  T_e_SG_D_1 : Outport  Port=3
  w_SG_D_1_out : Outport  Port=4
  theta_SG_D_1_out : Outport  Port=5
  wires:
  d_Px_1_SG_D_1_block/1(Blockout_d_Px_1_SG_D_1_85706) -> Px_1_SG_D_1/1
  V_f_SG_D_1/1 -> d_V_f_SG_D_1_block/14(State_V_f_SG_D_1_75aeb), d_E_fd_SG_D_1_block/2(State_V_f_SG_D_1_f4af9)
  psi_kq_SG_D_1/1 -> d_psi_q_SG_D_1_block/2(State_psi_kq_SG_D_1_7a833), d_psi_gq_SG_D_1_block/3(State_psi_kq_SG_D_1_40a2b), d_psi_gq_SG_D_1_block/5(State_psi_kq_SG_D_1_b9c48), d_psi_kq_SG_D_1_block/2(State_psi_kq_SG_D_1_e8a00), d_psi_kq_SG_D_1_block/4(State_psi_kq_SG_D_1_7c8e1), d_w_SG_D_1_block/5(State_psi_kq_SG_D_1_82b32), d_psi_gq_SG_D_1_block/8(State_psi_kq_SG_D_1_a5785), d_V_f_SG_D_1_block/10(State_psi_kq_SG_D_1_ae2e4), i_q_SG_D_1_block/2(State_psi_kq_SG_D_1_d3167), T_e_SG_D_1_block/3(State_psi_kq_SG_D_1_a4a45), i_d_SG_D_1_block/2(State_psi_kq_SG_D_1_c101c)
  w_SG_D_1_out_block/1(Blockout_w_SG_D_1_out_7bd8a) -> w_SG_D_1_out/1
  d_theta_SG_D_1_block/1(Blockout_d_theta_SG_D_1_084ed) -> theta_SG_D_1/1
  w_SG_D_1/1 -> d_psi_d_SG_D_1_block/9(State_w_SG_D_1_1bb72), d_psi_q_SG_D_1_block/9(State_w_SG_D_1_70743), d_V_f_SG_D_1_block/8(State_w_SG_D_1_bf45e), d_w_SG_D_1_block/1(State_w_SG_D_1_c5caf), d_V_f_SG_D_1_block/13(State_w_SG_D_1_c7aef), d_T_m_SG_D_1_block/1(State_w_SG_D_1_e7a7d), d_Px_1_SG_D_1_block/2(State_w_SG_D_1_3979b), d_Px_3_SG_D_1_block/6(State_w_SG_D_1_734a8), w_SG_D_1_out_block/1(State_w_SG_D_1_ada09), d_theta_SG_D_1_block/1(State_w_SG_D_1_12e76), d_Px_2_SG_D_1_block/4(State_w_SG_D_1_c572b)
  d_Px_3_SG_D_1_block/1(Blockout_d_Px_3_SG_D_1_28941) -> Px_3_SG_D_1/1
  d_Px_2_SG_D_1_block/1(Blockout_d_Px_2_SG_D_1_8a1c6) -> Px_2_SG_D_1/1
  d_T_m_SG_D_1_block/1(Blockout_d_T_m_SG_D_1_655fc) -> T_m_SG_D_1/1
  psi_gq_SG_D_1/1 -> d_psi_q_SG_D_1_block/1(State_psi_gq_SG_D_1_86fd1), d_psi_gq_SG_D_1_block/1(State_psi_gq_SG_D_1_c686b), d_psi_gq_SG_D_1_block/2(State_psi_gq_SG_D_1_65a16), d_psi_gq_SG_D_1_block/7(State_psi_gq_SG_D_1_8bc70), d_psi_kq_SG_D_1_block/1(State_psi_gq_SG_D_1_d81e0), d_psi_gq_SG_D_1_block/4(State_psi_gq_SG_D_1_462c5), d_V_f_SG_D_1_block/9(State_psi_gq_SG_D_1_51f29), i_d_SG_D_1_block/1(State_psi_gq_SG_D_1_bd1f3), i_q_SG_D_1_block/1(State_psi_gq_SG_D_1_ce74b), d_psi_kq_SG_D_1_block/3(State_psi_gq_SG_D_1_5f22b), d_w_SG_D_1_block/4(State_psi_gq_SG_D_1_fd6cf), T_e_SG_D_1_block/2(State_psi_gq_SG_D_1_f0c91)
  psi_fd_SG_D_1/1 -> d_psi_fd_SG_D_1_block/2(State_psi_fd_SG_D_1_400c1), d_psi_fd_SG_D_1_block/4(State_psi_fd_SG_D_1_b6078), d_psi_fd_SG_D_1_block/7(State_psi_fd_SG_D_1_0fece), d_psi_fd_SG_D_1_block/10(State_psi_fd_SG_D_1_f7919), d_psi_d_SG_D_1_block/3(State_psi_fd_SG_D_1_6a197), d_psi_1d_SG_D_1_block/5(State_psi_fd_SG_D_1_34365), d_psi_1d_SG_D_1_block/2(State_psi_fd_SG_D_1_45ba0), d_w_SG_D_1_block/10(State_psi_fd_SG_D_1_8c12b), d_V_f_SG_D_1_block/6(State_psi_fd_SG_D_1_3f25c), i_q_SG_D_1_block/7(State_psi_fd_SG_D_1_7f858), i_d_SG_D_1_block/7(State_psi_fd_SG_D_1_58188), T_e_SG_D_1_block/8(State_psi_fd_SG_D_1_11963)
  Px_2_SG_D_1/1 -> d_Px_3_SG_D_1_block/3(State_Px_2_SG_D_1_7f631), d_Px_2_SG_D_1_block/1(State_Px_2_SG_D_1_37bd3), d_Px_3_SG_D_1_block/2(State_Px_2_SG_D_1_d417b)
  d_E_fd_SG_D_1_block/1(Blockout_d_E_fd_SG_D_1_5e902) -> E_fd_SG_D_1/1
  psi_1d_SG_D_1/1 -> d_psi_fd_SG_D_1_block/3(State_psi_1d_SG_D_1_b4278), d_psi_fd_SG_D_1_block/5(State_psi_1d_SG_D_1_5bc63), d_psi_fd_SG_D_1_block/8(State_psi_1d_SG_D_1_00684), d_psi_d_SG_D_1_block/1(State_psi_1d_SG_D_1_fda93), d_psi_1d_SG_D_1_block/3(State_psi_1d_SG_D_1_6ec63), d_w_SG_D_1_block/8(State_psi_1d_SG_D_1_82e43), d_psi_1d_SG_D_1_block/1(State_psi_1d_SG_D_1_12b31), d_V_f_SG_D_1_block/4(State_psi_1d_SG_D_1_19aff), i_d_SG_D_1_block/5(State_psi_1d_SG_D_1_84ef0), i_q_SG_D_1_block/5(State_psi_1d_SG_D_1_f658e), T_e_SG_D_1_block/6(State_psi_1d_SG_D_1_a3712)
  psi_d_SG_D_1/1 -> d_psi_fd_SG_D_1_block/6(State_psi_d_SG_D_1_ec64c), d_psi_fd_SG_D_1_block/9(State_psi_d_SG_D_1_6472c), d_psi_d_SG_D_1_block/2(State_psi_d_SG_D_1_4a637), d_psi_q_SG_D_1_block/8(State_psi_d_SG_D_1_f3a29), d_psi_1d_SG_D_1_block/4(State_psi_d_SG_D_1_0b6f3), d_V_f_SG_D_1_block/12(State_psi_d_SG_D_1_12547), i_d_SG_D_1_block/6(State_psi_d_SG_D_1_be19d), d_w_SG_D_1_block/9(State_psi_d_SG_D_1_4b6c5), d_w_SG_D_1_block/3(State_psi_d_SG_D_1_1f625), i_q_SG_D_1_block/6(State_psi_d_SG_D_1_fbe87), T_e_SG_D_1_block/7(State_psi_d_SG_D_1_8fbb1), d_V_f_SG_D_1_block/5(State_psi_d_SG_D_1_925b9), T_e_SG_D_1_block/1(State_psi_d_SG_D_1_90645)
  theta_SG_D_1/1 -> d_psi_d_SG_D_1_block/5(State_theta_SG_D_1_66e05), d_psi_q_SG_D_1_block/5(State_theta_SG_D_1_2d0e9), d_psi_q_SG_D_1_block/7(State_theta_SG_D_1_d049a), i_d_SG_D_1_block/4(State_theta_SG_D_1_50d30), d_psi_d_SG_D_1_block/7(State_theta_SG_D_1_b6b51), i_d_SG_D_1_block/8(State_theta_SG_D_1_75ccd), i_q_SG_D_1_block/4(State_theta_SG_D_1_527e7), i_q_SG_D_1_block/8(State_theta_SG_D_1_42a46), theta_SG_D_1_out_block/1(State_theta_SG_D_1_cade5)
  T_m_SG_D_1/1 -> d_T_m_SG_D_1_block/2(State_T_m_SG_D_1_599df), d_w_SG_D_1_block/2(State_T_m_SG_D_1_31f02)
  v_d_SG_D_1/1 -> d_psi_d_SG_D_1_block/4(Input_v_d_SG_D_1_eef26), d_psi_q_SG_D_1_block/4(Input_v_d_SG_D_1_1af0c)
  v_q_SG_D_1/1 -> d_psi_d_SG_D_1_block/6(Input_v_q_SG_D_1_363cd), d_psi_q_SG_D_1_block/6(Input_v_q_SG_D_1_f6700)
  Px_1_SG_D_1/1 -> d_Px_1_SG_D_1_block/1(State_Px_1_SG_D_1_50cb8), d_Px_2_SG_D_1_block/2(State_Px_1_SG_D_1_cd8bf), d_Px_2_SG_D_1_block/3(State_Px_1_SG_D_1_d048c), d_Px_3_SG_D_1_block/4(State_Px_1_SG_D_1_53e62), d_Px_3_SG_D_1_block/5(State_Px_1_SG_D_1_57d0c)
  psi_q_SG_D_1/1 -> d_psi_d_SG_D_1_block/8(State_psi_q_SG_D_1_30b1b), d_psi_q_SG_D_1_block/3(State_psi_q_SG_D_1_9717c), d_psi_gq_SG_D_1_block/6(State_psi_q_SG_D_1_39993), d_psi_gq_SG_D_1_block/9(State_psi_q_SG_D_1_ce386), d_psi_kq_SG_D_1_block/5(State_psi_q_SG_D_1_9c6bf), d_w_SG_D_1_block/7(State_psi_q_SG_D_1_e2524), d_V_f_SG_D_1_block/7(State_psi_q_SG_D_1_d643a), i_d_SG_D_1_block/3(State_psi_q_SG_D_1_779e3), d_V_f_SG_D_1_block/11(State_psi_q_SG_D_1_20da0), d_w_SG_D_1_block/6(State_psi_q_SG_D_1_4134d), i_q_SG_D_1_block/3(State_psi_q_SG_D_1_d260e), T_e_SG_D_1_block/5(State_psi_q_SG_D_1_ce309), T_e_SG_D_1_block/4(State_psi_q_SG_D_1_cd1a7)
  d_V_f_SG_D_1_block/1(Blockout_d_V_f_SG_D_1_31ba3) -> V_f_SG_D_1/1
  d_R_f_SG_D_1_block/1(Blockout_d_R_f_SG_D_1_7e349) -> R_f_SG_D_1/1
  d_psi_kq_SG_D_1_block/1(Blockout_d_psi_kq_SG_D_1_2025a) -> psi_kq_SG_D_1/1
  T_e_SG_D_1_block/1(Blockout_T_e_SG_D_1_47b6a) -> T_e_SG_D_1/1
  d_psi_gq_SG_D_1_block/1(Blockout_d_psi_gq_SG_D_1_0214b) -> psi_gq_SG_D_1/1
  i_d_SG_D_1_block/1(Blockout_i_d_SG_D_1_acf57) -> i_d_SG_D_1/1
  i_q_SG_D_1_block/1(Blockout_i_q_SG_D_1_ba4c2) -> i_q_SG_D_1/1
  d_psi_1d_SG_D_1_block/1(Blockout_d_psi_1d_SG_D_1_a7c17) -> psi_1d_SG_D_1/1
  d_psi_q_SG_D_1_block/1(Blockout_d_psi_q_SG_D_1_385db) -> psi_q_SG_D_1/1
  d_w_SG_D_1_block/1(Blockout_d_w_SG_D_1_527e8) -> w_SG_D_1/1
  d_psi_d_SG_D_1_block/1(Blockout_d_psi_d_SG_D_1_63859) -> psi_d_SG_D_1/1
  theta_SG_D_1_out_block/1(Blockout_theta_SG_D_1_out_6277a) -> theta_SG_D_1_out/1
  Px_3_SG_D_1/1 -> d_V_f_SG_D_1_block/3(State_Px_3_SG_D_1_a16d6), d_Px_3_SG_D_1_block/1(State_Px_3_SG_D_1_043cf)
  R_f_SG_D_1/1 -> d_V_f_SG_D_1_block/2(State_R_f_SG_D_1_bb479), d_R_f_SG_D_1_block/2(State_R_f_SG_D_1_dffc8)
  E_fd_SG_D_1/1 -> d_R_f_SG_D_1_block/1(State_E_fd_SG_D_1_563f1), d_E_fd_SG_D_1_block/1(State_E_fd_SG_D_1_1c8d2), d_psi_fd_SG_D_1_block/1(State_E_fd_SG_D_1_fed90), d_V_f_SG_D_1_block/1(State_E_fd_SG_D_1_f00c0)
  d_psi_fd_SG_D_1_block/1(Blockout_d_psi_fd_SG_D_1_78404) -> psi_fd_SG_D_1/1
